simulink model "uz_3ph_ParameterID"  (R2022b)
settings: Solver=FixedStepDiscrete  StartTime=0.0  StopTime=160  FixedStep=0.000005  RelTol=1e-3  EnableMultiTasking=on
model workspace (MATLAB code in the model file):
  | cmdLim = Simulink.Parameter;
  | cmdLim.Value = 15;
  | cmdLim.Description = 'Limit for controlling the maximum surface command angle.';
  | cmdLim.Min = 0;
  | cmdLim.Max = 90;
  | cmdLim.DocUnits = 'deg';
  | 
  | dispGain = Simulink.Parameter;
  | dispGain.Value = 0.75;
  | dispGain.Description = 'Gain applied to the displacement error.';
  | dispGain.Min = 0;
  | dispGain.Max = [];
  | dispGain.DocUnits = 'deg/sec/deg';
  | 
  | dispLim = Simulink.Parameter;
  | dispLim.Value = 30;
  | dispLim.Description = 'Limit for controlling the maximum commanded angle.';
  | dispLim.Min = 0;
  | dispLim.Max = 180;
  | dispLim.DocUnits = 'deg';
  | 
  | intGain = Simulink.Parameter;
  | intGain.Value = 0.5;
  | intGain.Description = 'Gain applied to the integral error.';
  | intGain.Min = 0;
  | intGain.Max = [];
  | intGain.DocUnits = 'deg/sec/deg/sec';
  | 
  | intLim = Simulink.Parameter;
  | intLim.Value = 5;
  | intLim.Description = 'Limit for controlling the maximum commanded angle.';
  | intLim.Min = 0;
  | intLim.Max = 90;
  | intLim.DocUnits = 'deg';
  | 
  | rateGain = Simulink.Parameter;
  | rateGain.Value = 2;
  | rateGain.Description = 'Gain applied to the rate error.';
  | rateGain.Min = 0;
  | rateGain.Max = [];
  | rateGain.DocUnits = 'deg/deg/sec';
  | 
  | rateLim = Simulink.Parameter;
  | rateLim.Value = 6;
  | rateLim.Description = 'Limit for controlling the maximum commanded angle.';
  | rateLim.Min = 0;
  | rateLim.Max = 180;
  | rateLim.DocUnits = 'deg/sec';
  | 
  | hdgGain = Simulink.Parameter;
  | hdgGain.Value = 0.015;
values from neighbouring files (symbols this model uses):
  d_d_TMS = 0.005    [Parameter_Init_Buehler_201.m]
  d_f_hardware = 200000    [Parameter_Init_Buehler_201.m]
  d_f_states = 20000    [Parameter_Init_Buehler_201.m]
  d_i_max = 15    [Parameter_Init_Buehler_201.m]
  d_i_min = -d_i_max    (= -15)    [Parameter_Init_Buehler_201.m]
  d_I_n = 8    [Parameter_Init_Buehler_201.m]
  d_J_Coupling_M_E = 2e-6    (= 2e-06)    [Parameter_Init_Buehler_201.m]
  d_J_Coupling_M_Ms = 2e-20    [Parameter_Init_Buehler_201.m]
  d_J_Ms_L = d_J_Ms_M    (= 1.26363648e-05)    [Parameter_Init_Buehler_201.m]
  d_J_Ms_M = 0.5*0.5*((0.5*d_d_Ms)^4)*3.14*d_l_Ms*d_rho_Ms    (= 1.26363648e-05)    [Parameter_Init_Buehler_201.m]
  d_L_d = 0.00031    [Parameter_Init_Buehler_201.m]
  d_L_q = 0.00033    [Parameter_Init_Buehler_201.m]
  d_p = 4    [Parameter_Init_Buehler_201.m]
  d_psi_pm = 0.0075    [Parameter_Init_Buehler_201.m]
  d_R_ph = d_R_ph_ph/2    (= 0.089)    [Parameter_Init_Buehler_201.m]
  d_y_max = 10    [Parameter_Init_Buehler_201.m]
  d_y_min = -d_y_max    (= -10)    [Parameter_Init_Buehler_201.m]
undefined symbols (not defined in the file or in its folder): i_dq, i_dq_ref, n_ref, V_abc, v_dq
libraries: fl_lib x47, nesl_utility x30, ee_lib x18, simulink x8, spsabctodq0Lib x2, spsdq0toabcLib x1, spsTriangleGeneratorLib x1
(part 3 of 4)

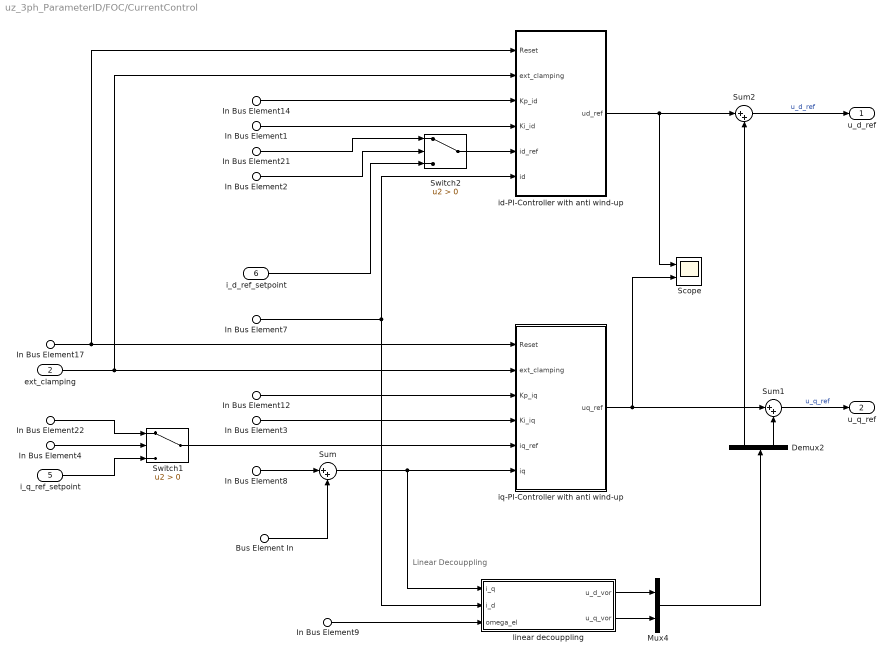
== system uz_3ph_ParameterID/FOC/CurrentControl ==
  note: Linear Decouppling
  Bus Element In : Inport  PortName=TwoMassID_output  Element=PRBS_out
  ext_clamping : Inport  Port=2
  In Bus Element1 : Inport  Port=3  PortName=FOC_State_outputs  Element=Ki_id_out
  In Bus Element14 : Inport  Port=3  PortName=FOC_State_outputs  Element=Kp_id_out
  In Bus Element2 : Inport  Port=3  PortName=FOC_State_outputs  Element=enableFOC_current
  In Bus Element4 : Inport  Port=3  PortName=FOC_State_outputs  Element=enableFOC_current
  In Bus Element21 : Inport  Port=3  PortName=FOC_State_outputs  Element=i_dq_ref.d
  In Bus Element22 : Inport  Port=3  PortName=FOC_State_outputs  Element=i_dq_ref.q
  In Bus Element17 : Inport  Port=3  PortName=FOC_State_outputs  Element=resetIntegrator
  In Bus Element12 : Inport  Port=3  PortName=FOC_State_outputs  Element=Kp_iq_out
  In Bus Element3 : Inport  Port=3  PortName=FOC_State_outputs  Element=Ki_iq_out
  In Bus Element9 : Inport  Port=4  PortName=ActualValues  Element=omega_el
  In Bus Element7 : Inport  Port=4  PortName=ActualValues  Element=i_dq.d
  In Bus Element8 : Inport  Port=4  PortName=ActualValues  Element=i_dq.q
  i_q_ref_setpoint : Inport  Port=5
  i_d_ref_setpoint : Inport  Port=6
  Demux2 : Demux  Outputs=2
  Mux4 : Mux  Inputs=2
  Scope : Scope  NumInputPorts=2
  Sum : Sum  Inputs=|++
  Sum1 : Sum  Inputs=|++
  Sum2 : Sum  Inputs=|++
  Switch1 : Switch  Criteria=u2 > Threshold  SaturateOnIntegerOverflow=off  InputSameDT=off
  Switch2 : Switch  Criteria=u2 > Threshold  SaturateOnIntegerOverflow=off  InputSameDT=off
  id-PI-Controller with anti wind-up : Subsystem
  iq-PI-Controller with anti wind-up : Subsystem
  linear decouppling : Subsystem
  u_d_ref : Outport  OutDataTypeStr=single
  u_q_ref : Outport  Port=2  OutDataTypeStr=single
  wires:
  In Bus Element7/1 -> id-PI-Controller with anti wind-up/6(id), linear decouppling/2(i_d)
  In Bus Element1/1 -> id-PI-Controller with anti wind-up/4(Ki_id)
  Sum/1 -> linear decouppling/1(i_q), iq-PI-Controller with anti wind-up/6(iq)
  In Bus Element3/1 -> iq-PI-Controller with anti wind-up/4(Ki_iq)
  In Bus Element14/1 -> id-PI-Controller with anti wind-up/3(Kp_id)
  In Bus Element12/1 -> iq-PI-Controller with anti wind-up/3(Kp_iq)
  In Bus Element17/1 -> iq-PI-Controller with anti wind-up/1(Reset), id-PI-Controller with anti wind-up/1(Reset)
  Switch1/1 -> iq-PI-Controller with anti wind-up/5(iq_ref)
  ext_clamping/1 -> iq-PI-Controller with anti wind-up/2(ext_clamping), id-PI-Controller with anti wind-up/2(ext_clamping)
  In Bus Element9/1 -> linear decouppling/3(omega_el)
  Mux4/1 -> Demux2/1
  linear decouppling/1(u_d_vor) -> Mux4/1
  linear decouppling/2(u_q_vor) -> Mux4/2
  Demux2/2 -> Sum1/2
  iq-PI-Controller with anti wind-up/1(uq_ref) -> Scope/2, Sum1/1
  id-PI-Controller with anti wind-up/1(ud_ref) -> Scope/1, Sum2/1
  Demux2/1 -> Sum2/2
  Sum1/1 -> u_q_ref/1  "u_q_ref"
  In Bus Element22/1 -> Switch1/1
  In Bus Element4/1 -> Switch1/2
  i_q_ref_setpoint/1 -> Switch1/3
  Sum2/1 -> u_d_ref/1  "u_d_ref"
  In Bus Element21/1 -> Switch2/1
  i_d_ref_setpoint/1 -> Switch2/3
  Switch2/1 -> id-PI-Controller with anti wind-up/5(id_ref)
  In Bus Element2/1 -> Switch2/2
  In Bus Element8/1 -> Sum/1
  Bus Element In/1 -> Sum/2

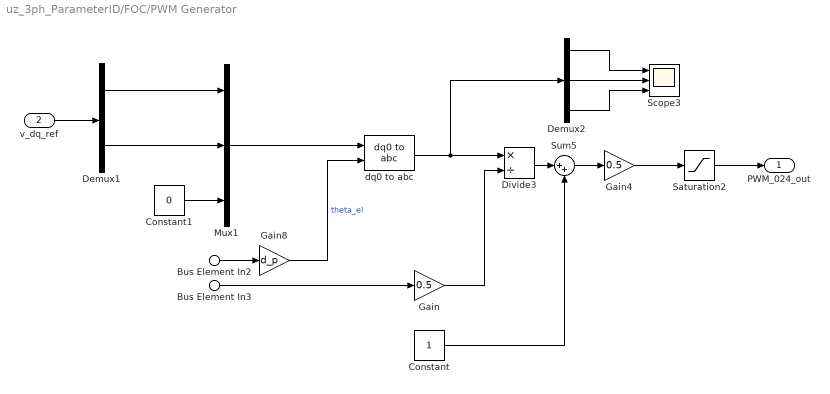
== system uz_3ph_ParameterID/FOC/PWM Generator ==
  Bus Element In2 : Inport  PortName=ActualValues  Element=theta_m
  Bus Element In3 : Inport  PortName=ActualValues  Element=V_DC
  v_dq_ref : Inport  Port=2
  Constant : Constant  OutDataTypeStr=single
  Constant1 : Constant  Value=0  OutDataTypeStr=single
  Demux1 : Demux  Outputs=2
  Demux2 : Demux  Outputs=3
  Divide3 : Product  Inputs=*/
  Gain : Gain  Gain=0.5
  Gain4 : Gain  Gain=0.5
  Gain8 : Gain  Gain=d_p  OutDataTypeStr=single
  Mux1 : Mux  Inputs=3
  Saturation2 : Saturate  UpperLimit=1  LowerLimit=0
  Scope3 : Scope  NumInputPorts=3
  Sum5 : Sum  Inputs=|++
  dq0 to abc : spsdq0toabcLib/dq0 to abc  Alignment=Aligned with phase A axis
  PWM_024_out : Outport  VectorParamsAs1DForOutWhenUnconnected=off
  wires:
  Constant/1 -> Sum5/2
  Demux2/2 -> Scope3/2
  Gain4/1 -> Saturation2/1
  Demux2/1 -> Scope3/1
  Demux2/3 -> Scope3/3
  Gain/1 -> Divide3/2
  Sum5/1 -> Gain4/1
  Mux1/1 -> dq0 to abc/1
  dq0 to abc/1 -> Demux2/1, Divide3/1
  Divide3/1 -> Sum5/1
  Bus Element In3/1 -> Gain/1
  Constant1/1 -> Mux1/3
  Demux1/2 -> Mux1/2
  Saturation2/1 -> PWM_024_out/1
  v_dq_ref/1 -> Demux1/1
  Demux1/1 -> Mux1/1
  Bus Element In2/1 -> Gain8/1
  Gain8/1 -> dq0 to abc/2  "theta_el"

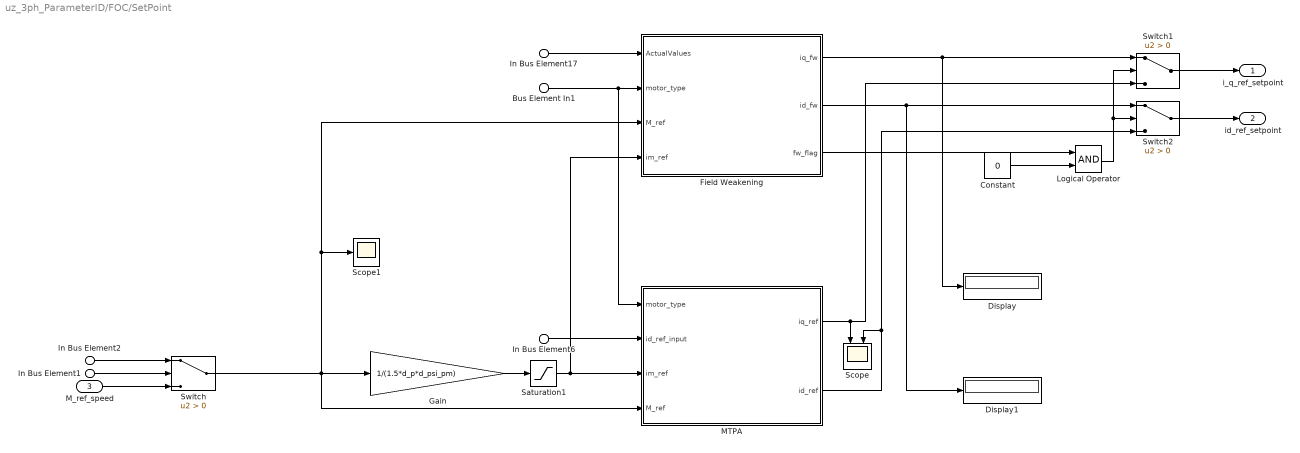
== system uz_3ph_ParameterID/FOC/SetPoint ==
  In Bus Element17 : Inport  PortName=ActualValues
  In Bus Element6 : Inport  Port=2  PortName=FOC_State_outputs  Element=i_dq_ref.d
  In Bus Element1 : Inport  Port=2  PortName=FOC_State_outputs  Element=enableFOC_torque
  In Bus Element2 : Inport  Port=2  PortName=FOC_State_outputs  Element=M_ref_FOC
  M_ref_speed : Inport  Port=3
  Bus Element In1 : Inport  Port=4  PortName=GlobalConfig  Element=motor_type
  Constant : Constant  Value=0
  Display : Display
  Display1 : Display
  Field Weakening : Subsystem
  Gain : Gain  Gain=1/(1.5*d_p*d_psi_pm)
  Logical Operator : Logic  AllPortsSameDT=off  OutDataTypeStr=boolean
  MTPA : Subsystem
  Saturation1 : Saturate  UpperLimit=d_i_max  LowerLimit=d_i_min
  Scope : Scope  NumInputPorts=2
  Scope1 : Scope
  Switch : Switch  Criteria=u2 > Threshold  SaturateOnIntegerOverflow=off  InputSameDT=off
  Switch1 : Switch  Criteria=u2 > Threshold  SaturateOnIntegerOverflow=off  InputSameDT=off
  Switch2 : Switch  Criteria=u2 > Threshold  SaturateOnIntegerOverflow=off  InputSameDT=off
  i_q_ref_setpoint : Outport  OutDataTypeStr=single
  id_ref_setpoint : Outport  Port=2  OutDataTypeStr=single
  wires:
  In Bus Element17/1 -> Field Weakening/1(ActualValues)
  Bus Element In1/1 -> MTPA/1(motor_type), Field Weakening/2(motor_type)
  In Bus Element6/1 -> MTPA/2(id_ref_input)
  MTPA/1(iq_ref) -> Switch1/3, Scope/1
  MTPA/2(id_ref) -> Switch2/3, Scope/2
  Switch2/1 -> id_ref_setpoint/1
  Field Weakening/2(id_fw) -> Display1/1, Switch2/1
  Saturation1/1 -> Field Weakening/4(im_ref), MTPA/3(im_ref)
  Field Weakening/1(iq_fw) -> Switch1/1, Display/1
  Logical Operator/1 -> Switch1/2, Switch2/2
  Gain/1 -> Saturation1/1
  Switch/1 -> Scope1/1, Field Weakening/3(M_ref), MTPA/4(M_ref), Gain/1
  Switch1/1 -> i_q_ref_setpoint/1
  Field Weakening/3(fw_flag) -> Logical Operator/1
  Constant/1 -> Logical Operator/2
  M_ref_speed/1 -> Switch/3
  In Bus Element1/1 -> Switch/2
  In Bus Element2/1 -> Switch/1

== system uz_3ph_ParameterID/FOC/SpeedControl ==
  ext_clamping : Inport
  In Bus Element7 : Inport  Port=2  PortName=FOC_State_outputs  Element=n_ref_FOC
  In Bus Element10 : Inport  Port=2  PortName=FOC_State_outputs  Element=resetIntegrator
  In Bus Element17 : Inport  Port=3  PortName=ActualValues  Element=omega_el
  Bus Element In1 : Inport  Port=4  PortName=GlobalConfig  Element=Ki_n
  Bus Element In : Inport  Port=4  PortName=GlobalConfig  Element=Kp_n
  Constant : Constant
  Constant1 : Constant  Value=-1
  Gain : Gain  Gain=1/d_p
  omega-PI-Controller with anti wind-up : Subsystem
  M_ref : Outport  OutDataTypeStr=single
  wires:
  In Bus Element10/1 -> omega-PI-Controller with anti wind-up/1(Reset)
  In Bus Element7/1 -> omega-PI-Controller with anti wind-up/5(n_ref_rpm)
  Bus Element In1/1 -> omega-PI-Controller with anti wind-up/4(Ki_n)
  Bus Element In/1 -> omega-PI-Controller with anti wind-up/3(Kp_n)
  ext_clamping/1 -> omega-PI-Controller with anti wind-up/2(ext_clamping)
  In Bus Element17/1 -> Gain/1
  omega-PI-Controller with anti wind-up/1(M_ref) -> M_ref/1
  Constant/1 -> omega-PI-Controller with anti wind-up/7(upper_limit)
  Constant1/1 -> omega-PI-Controller with anti wind-up/8(lower_limit)
  Gain/1 -> omega-PI-Controller with anti wind-up/6(omega)

== system uz_3ph_ParameterID/Hardware/Coupling Encoder ==
  note: 1) Add Subsystem or Model blocks as valid variant choices.
      | 2) You cannot connect blocks at this level. At simulation, connectivity is automatically
      | determined, based on the active variant and port name matching.
  Inertia : Subsystem  VariantControl=(default)
  Spring Damper System : Subsystem  VariantControl=TMS1
  Input : PMIOPort  Side=Left
  output : PMIOPort  Port=2  Side=Right

== system uz_3ph_ParameterID/Hardware/Measurement Shaft ==
  note: 1) Add Subsystem or Model blocks as valid variant choices.
      | 2) You cannot connect blocks at this level. At simulation, connectivity is automatically
      | determined, based on the active variant and port name matching.
  Spring Damper System : Subsystem  VariantControl=TMS1
  default : Subsystem  VariantControl=(default)
  Input : PMIOPort  Side=Left
  output : PMIOPort  Port=2  Side=Right

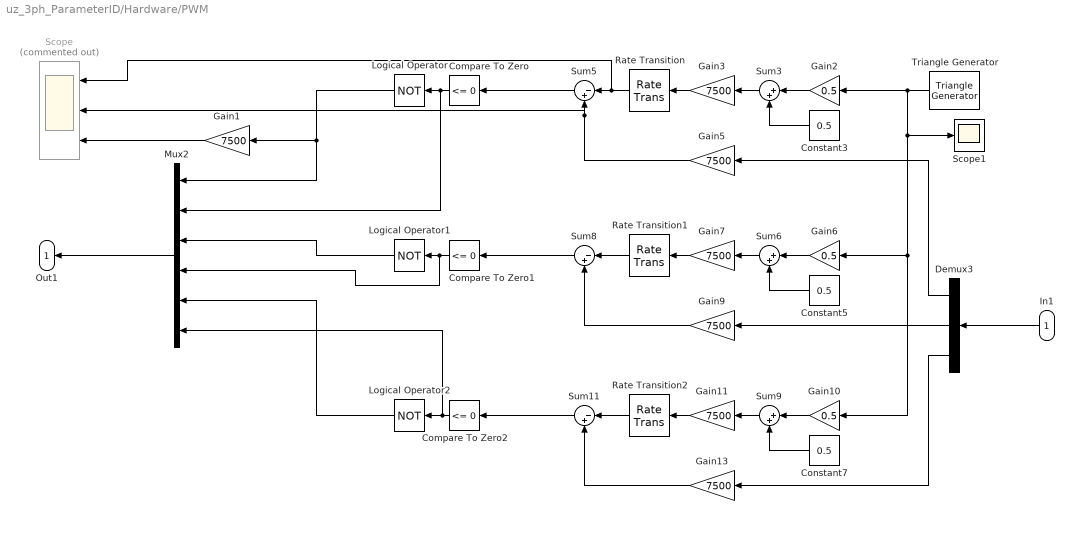
== system uz_3ph_ParameterID/Hardware/PWM ==
  In1 : Inport
  Compare To Zero : simulink/Logic and Bit Operations/Compare To Zero  relop=<=  OutDataTypeStr=boolean
  Compare To Zero1 : simulink/Logic and Bit Operations/Compare To Zero  relop=<=  OutDataTypeStr=boolean
  Compare To Zero2 : simulink/Logic and Bit Operations/Compare To Zero  relop=<=  OutDataTypeStr=boolean
  Constant3 : Constant  Value=0.5
  Constant5 : Constant  Value=0.5
  Constant7 : Constant  Value=0.5
  Demux3 : Demux  Outputs=3
  Gain{1,3,5,7,9,11,13} (7 alike) : Gain  Gain=7500  ParamDataTypeStr=single
  Gain10 : Gain  Gain=0.5
  Gain2 : Gain  Gain=0.5
  Gain6 : Gain  Gain=0.5
  Logical Operator : Logic  Operator=NOT  AllPortsSameDT=off  OutDataTypeStr=boolean
  Logical Operator1 : Logic  Operator=NOT  AllPortsSameDT=off  OutDataTypeStr=boolean
  Logical Operator2 : Logic  Operator=NOT  AllPortsSameDT=off  OutDataTypeStr=boolean
  Mux2 : Mux  Inputs=6
  Rate Transition : RateTransition  OutPortSampleTime=1/d_f_hardware
  Rate Transition1 : RateTransition  OutPortSampleTime=1/d_f_hardware
  Rate Transition2 : RateTransition  OutPortSampleTime=1/d_f_hardware
  Scope : Scope  Commented=on  NumInputPorts=3
  Scope1 : Scope
  Sum11 : Sum  Inputs=|-+
  Sum3 : Sum  Inputs=|++
  Sum5 : Sum  Inputs=|-+
  Sum6 : Sum  Inputs=|++
  Sum8 : Sum  Inputs=|-+
  Sum9 : Sum  Inputs=|++
  Triangle Generator : spsTriangleGeneratorLib/Triangle Generator  Freq=10000  Phase=0  Ts=1/d_f_hardware
  Out1 : Outport  VectorParamsAs1DForOutWhenUnconnected=off
  wires:
  Demux3/3 -> Gain13/1
  Logical Operator2/1 -> Mux2/5
  Logical Operator1/1 -> Mux2/3
  Mux2/1 -> Out1/1
  Compare To Zero2/1 -> Mux2/6, Logical Operator2/1
  Gain10/1 -> Sum9/1
  Sum8/1 -> Compare To Zero1/1
  Gain6/1 -> Sum6/1
  Sum9/1 -> Gain11/1
  Triangle Generator/1 -> Scope1/1, Gain10/1, Gain6/1, Gain2/1
  Sum6/1 -> Gain7/1
  Demux3/2 -> Gain9/1
  Compare To Zero1/1 -> Mux2/4, Logical Operator1/1
  Constant5/1 -> Sum6/2
  Constant7/1 -> Sum9/2
  Sum11/1 -> Compare To Zero2/1
  Sum3/1 -> Gain3/1
  Constant3/1 -> Sum3/2
  Demux3/1 -> Gain5/1
  Sum5/1 -> Compare To Zero/1
  Gain2/1 -> Sum3/1
  In1/1 -> Demux3/1
  Gain3/1 -> Rate Transition/1
  Gain7/1 -> Rate Transition1/1
  Gain11/1 -> Rate Transition2/1
  Gain5/1 -> Scope/2, Sum5/2
  Gain9/1 -> Sum8/2
  Gain13/1 -> Sum11/2
  Rate Transition/1 -> Scope/1, Sum5/1
  Rate Transition1/1 -> Sum8/1
  Rate Transition2/1 -> Sum11/1
  Logical Operator/1 -> Gain1/1, Mux2/1
  Compare To Zero/1 -> Mux2/2, Logical Operator/1
  Gain1/1 -> Scope/3

== system uz_3ph_ParameterID/Hardware/Switch f. TMS ==
  note: 1) Add Subsystem or Model blocks as valid variant choices.
      | 2) You cannot connect blocks at this level. At simulation, connectivity is automatically
      | determined, based on the active variant and port name matching.
  closed : Subsystem  VariantControl=d_KupplZus==1
  open : Subsystem  VariantControl=d_KupplZus==0
  Input : PMIOPort  Side=Left
  output : PMIOPort  Port=2  Side=Right

== system uz_3ph_ParameterID/Hardware/coupling m. shaft ==
  note: 1) Add Subsystem or Model blocks as valid variant choices.
      | 2) You cannot connect blocks at this level. At simulation, connectivity is automatically
      | determined, based on the active variant and port name matching.
  Inertia : Subsystem  VariantControl=(default)
  Spring Damper System : Subsystem  VariantControl=TMS1
  Input : PMIOPort  Side=Left
  output : PMIOPort  Port=2  Side=Right

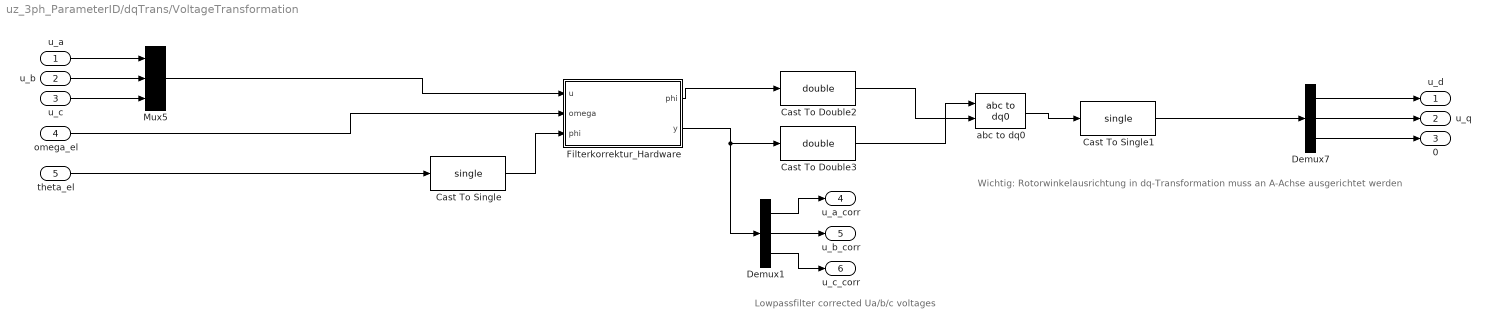
== system uz_3ph_ParameterID/dqTrans/VoltageTransformation ==
  note: Lowpassfilter corrected Ua/b/c voltages
  note: Wichtig: Rotorwinkelausrichtung in dq-Transformation
      | muss an A-Achse ausgerichtet werden
  u_a : Inport
  u_b : Inport  Port=2
  u_c : Inport  Port=3
  omega_el : Inport  Port=4
  theta_el : Inport  Port=5
  Cast To Double2 : DataTypeConversion  OutDataTypeStr=double  SaturateOnIntegerOverflow=off  RndMeth=Floor
  Cast To Double3 : DataTypeConversion  OutDataTypeStr=double  SaturateOnIntegerOverflow=off  RndMeth=Floor
  Cast To Single : DataTypeConversion  OutDataTypeStr=single  SaturateOnIntegerOverflow=off  RndMeth=Floor
  Cast To Single1 : DataTypeConversion  OutDataTypeStr=single  SaturateOnIntegerOverflow=off  RndMeth=Floor
  Demux1 : Demux  Outputs=3
  Demux7 : Demux  Outputs=3
  Filterkorrektur_Hardware : MATLAB Function  TreatAsAtomicUnit=on
  Mux5 : Mux  Inputs=3
  abc to dq0 : spsabctodq0Lib/abc to dq0  Alignment=Aligned with phase A axis
  u_d : Outport  VectorParamsAs1DForOutWhenUnconnected=off
  u_q : Outport  Port=2  VectorParamsAs1DForOutWhenUnconnected=off
  0 : Outport  Port=3  VectorParamsAs1DForOutWhenUnconnected=off
  u_a_corr : Outport  Port=4  VectorParamsAs1DForOutWhenUnconnected=off
  u_b_corr : Outport  Port=5  VectorParamsAs1DForOutWhenUnconnected=off
  u_c_corr : Outport  Port=6  VectorParamsAs1DForOutWhenUnconnected=off
  wires:
  abc to dq0/1 -> Cast To Single1/1
  Cast To Single1/1 -> Demux7/1
  Cast To Double3/1 -> abc to dq0/1
  Filterkorrektur_Hardware/2(y) -> Demux1/1, Cast To Double3/1
  Cast To Double2/1 -> abc to dq0/2
  Filterkorrektur_Hardware/1(phi) -> Cast To Double2/1
  Demux7/2 -> u_q/1
  Demux7/3 -> 0/1
  u_b/1 -> Mux5/2
  u_c/1 -> Mux5/3
  u_a/1 -> Mux5/1
  omega_el/1 -> Filterkorrektur_Hardware/2(omega)
  Mux5/1 -> Filterkorrektur_Hardware/1(u)
  theta_el/1 -> Cast To Single/1
  Cast To Single/1 -> Filterkorrektur_Hardware/3("phi ")
  Demux7/1 -> u_d/1
  Demux1/1 -> u_a_corr/1
  Demux1/2 -> u_b_corr/1
  Demux1/3 -> u_c_corr/1

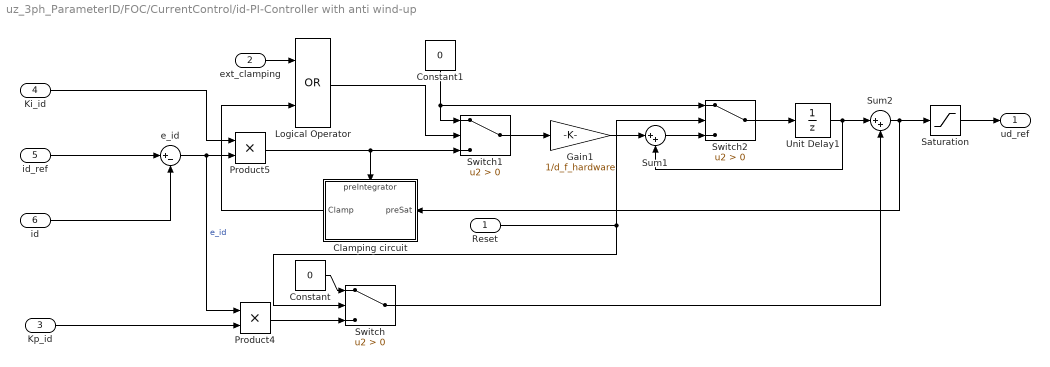
== system uz_3ph_ParameterID/FOC/CurrentControl/id-PI-Controller with anti wind-up ==
  Reset : Inport
  ext_clamping : Inport  Port=2
  Kp_id : Inport  Port=3
  Ki_id : Inport  Port=4
  id_ref : Inport  Port=5
  id : Inport  Port=6
  Clamping circuit : Subsystem
      settings: PortSchema="{\"entries\":[{\"content\":{\"sides\":[{\"content\":{\"connectorIds\":[\"In1\"]},\"type\":\"ConnectorPlacement.EquallySpacedRectSide\",\"uuid\":\"9b5eb3d3-336d-4b55-a615-0420b1cf4a48\"},{\"content\":{\"connectorIds\":[\"Out1\"],\"side\":\"RIGHT\"},\"type\":\"ConnectorPlacement.EquallySpacedRectSide\",\"uuid\":\"a73559ab-79dd-4c84-b45a-6a43ba4812e9\"},{\"content\":{\"connectorIds\":[\"In2\"],\"side\":\"TOP\"},\"type\":\"ConnectorPlacement.EquallySpacedRectSide\",\"uuid\":\"82c30f31-c271-4a2b-89be-8686aa9e20f3\"}]},\"type\":\"ConnectorPlacement.EquallySpacedConnector\",\"uuid\":\"376d2fe4-39b3-495b-8d80-8756076e2730\"}],\"packageUris\":[\"http://schema.mathworks.com/mf0/Connector/R2020b\"],\"version\":\"1.0\"}"
  Constant : Constant  Value=0  SampleTime=1/d_f_hardware
  Constant1 : Constant  Value=0  SampleTime=1/d_f_hardware
  Gain1 : Gain  Gain=1/d_f_hardware
  Logical Operator : Logic  Operator=OR  AllPortsSameDT=off  OutDataTypeStr=boolean
  Product4 : Product
  Product5 : Product
  Saturation : Saturate  UpperLimit=d_y_max  LowerLimit=d_y_min
  Sum1 : Sum  Inputs=|++  OutDataTypeStr=single
  Sum2 : Sum  Inputs=|++  OutDataTypeStr=single
  Switch : Switch  Criteria=u2 > Threshold  SaturateOnIntegerOverflow=off  InputSameDT=off
  Switch1 : Switch  Criteria=u2 > Threshold  SaturateOnIntegerOverflow=off  InputSameDT=off
  Switch2 : Switch  Criteria=u2 > Threshold  SaturateOnIntegerOverflow=off  InputSameDT=off
  Unit Delay1 : UnitDelay  SampleTime=-1  HasFrameUpgradeWarning=on
  e_id : Sum  Inputs=|+-
  ud_ref : Outport
  wires:
  Unit Delay1/1 -> Sum2/1, Sum1/2
  Kp_id/1 -> Product4/2
  id_ref/1 -> e_id/1
  Ki_id/1 -> Product5/1
  id/1 -> e_id/2
  e_id/1 -> Product5/2, Product4/1  "e_id"
  Switch/1 -> Sum2/2
  Logical Operator/1 -> Switch1/2
  ext_clamping/1 -> Logical Operator/1
  Sum2/1 -> Saturation/1, Clamping circuit/1(preSat)
  Clamping circuit/1(Clamp) -> Logical Operator/2
  Product5/1 -> Switch1/3, Clamping circuit/2(preIntegrator)
  Saturation/1 -> ud_ref/1
  Constant/1 -> Switch/1
  Product4/1 -> Switch/3
  Gain1/1 -> Sum1/1
  Constant1/1 -> Switch2/1, Switch1/1
  Reset/1 -> Switch/2, Switch2/2
  Sum1/1 -> Switch2/3
  Switch2/1 -> Unit Delay1/1
  Switch1/1 -> Gain1/1

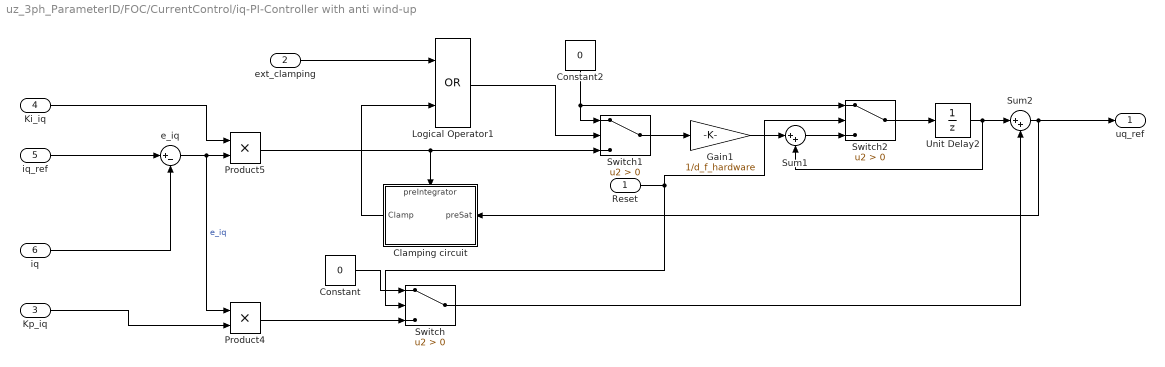
== system uz_3ph_ParameterID/FOC/CurrentControl/iq-PI-Controller with anti wind-up ==
  Reset : Inport
  ext_clamping : Inport  Port=2
  Kp_iq : Inport  Port=3
  Ki_iq : Inport  Port=4
  iq_ref : Inport  Port=5
  iq : Inport  Port=6
  Clamping circuit : Subsystem
      settings: PortSchema="{\"entries\":[{\"content\":{\"sides\":[{\"content\":{\"connectorIds\":[\"In1\"]},\"type\":\"ConnectorPlacement.EquallySpacedRectSide\",\"uuid\":\"9b5eb3d3-336d-4b55-a615-0420b1cf4a48\"},{\"content\":{\"connectorIds\":[\"Out1\"],\"side\":\"RIGHT\"},\"type\":\"ConnectorPlacement.EquallySpacedRectSide\",\"uuid\":\"a73559ab-79dd-4c84-b45a-6a43ba4812e9\"},{\"content\":{\"connectorIds\":[\"In2\"],\"side\":\"TOP\"},\"type\":\"ConnectorPlacement.EquallySpacedRectSide\",\"uuid\":\"82c30f31-c271-4a2b-89be-8686aa9e20f3\"}]},\"type\":\"ConnectorPlacement.EquallySpacedConnector\",\"uuid\":\"376d2fe4-39b3-495b-8d80-8756076e2730\"}],\"packageUris\":[\"http://schema.mathworks.com/mf0/Connector/R2020b\"],\"version\":\"1.0\"}"
  Constant : Constant  Value=0  SampleTime=1/d_f_hardware
  Constant2 : Constant  Value=0  SampleTime=1/d_f_hardware
  Gain1 : Gain  Gain=1/d_f_hardware
  Logical Operator1 : Logic  Operator=OR  AllPortsSameDT=off  OutDataTypeStr=boolean
  Product4 : Product
  Product5 : Product
  Sum1 : Sum  Inputs=|++  OutDataTypeStr=single
  Sum2 : Sum  Inputs=|++  OutDataTypeStr=single
  Switch : Switch  Criteria=u2 > Threshold  SaturateOnIntegerOverflow=off  InputSameDT=off
  Switch1 : Switch  Criteria=u2 > Threshold  SaturateOnIntegerOverflow=off  InputSameDT=off
  Switch2 : Switch  Criteria=u2 > Threshold  SaturateOnIntegerOverflow=off  InputSameDT=off
  Unit Delay2 : UnitDelay  SampleTime=-1  HasFrameUpgradeWarning=on
  e_iq : Sum  Inputs=|+-
  uq_ref : Outport
  wires:
  ext_clamping/1 -> Logical Operator1/1
  Kp_iq/1 -> Product4/2
  Ki_iq/1 -> Product5/1
  iq_ref/1 -> e_iq/1
  iq/1 -> e_iq/2
  e_iq/1 -> Product5/2, Product4/1  "e_iq"
  Unit Delay2/1 -> Sum2/1, Sum1/2
  Clamping circuit/1(Clamp) -> Logical Operator1/2
  Sum2/1 -> uq_ref/1, Clamping circuit/1(preSat)
  Switch/1 -> Sum2/2
  Constant/1 -> Switch/1
  Product4/1 -> Switch/3
  Switch2/1 -> Unit Delay2/1
  Gain1/1 -> Sum1/1
  Constant2/1 -> Switch2/1, Switch1/1
  Sum1/1 -> Switch2/3
  Product5/1 -> Switch1/3, Clamping circuit/2(preIntegrator)
  Switch1/1 -> Gain1/1
  Reset/1 -> Switch2/2, Switch/2
  Logical Operator1/1 -> Switch1/2

== system uz_3ph_ParameterID/FOC/CurrentControl/linear decouppling ==
  i_q : Inport
  i_d : Inport  Port=2
  omega_el : Inport  Port=3
  Gain : Gain  Gain=-d_L_q
  Gain4 : Gain  Gain=d_L_d
  Product : Product  SaturateOnIntegerOverflow=on
  Product1 : Product  SaturateOnIntegerOverflow=on
  Sum : Sum  Inputs=|++
  d_psi_pm : Constant  Value=d_psi_pm  OutDataTypeStr=Inherit: Inherit via back propagation  SampleTime=1/d_f_hardware
  u_d_vor : Outport  VectorParamsAs1DForOutWhenUnconnected=off
  u_q_vor : Outport  Port=2  VectorParamsAs1DForOutWhenUnconnected=off
  wires:
  i_q/1 -> Product/1
  Product1/1 -> u_q_vor/1
  Gain/1 -> Product/2
  Sum/1 -> Product1/1
  Product/1 -> u_d_vor/1
  omega_el/1 -> Gain/1, Product1/2
  Gain4/1 -> Sum/1
  d_psi_pm/1 -> Sum/2
  i_d/1 -> Gain4/1

== system uz_3ph_ParameterID/FOC/SetPoint/Field Weakening ==
  ActualValues : Inport  OutDataTypeStr=Bus: uz_ParaID_ActualValues_t
  motor_type : Inport  Port=2  OutDataTypeStr=uint16
  M_ref : Inport  Port=3  OutDataTypeStr=single
  im_ref : Inport  Port=4  OutDataTypeStr=single
  Constant : Constant  Value=d_R_ph  OutDataTypeStr=single
  Constant1 : Constant  Value=d_L_q  OutDataTypeStr=single
  Constant2 : Constant  Value=d_L_d  OutDataTypeStr=single
  Constant3 : Constant  Value=d_psi_pm  OutDataTypeStr=single
  Constant4 : Constant  Value=d_i_max  OutDataTypeStr=single
  Constant5 : Constant  Value=d_p  OutDataTypeStr=single
  Gain : Gain  Gain=60/(2*d_p*pi)
  MATLAB Function : MATLAB Function  TreatAsAtomicUnit=on
  n_cut in rpm : Display
  iq_fw : Outport  OutDataTypeStr=single
  id_fw : Outport  Port=2  OutDataTypeStr=single
  fw_flag : Outport  Port=3  OutDataTypeStr=boolean
  wires:
  Constant4/1 -> MATLAB Function/1(I_max)
  ActualValues/1 -> MATLAB Function/2(ActualValues)
  Constant/1 -> MATLAB Function/3(R)
  Constant1/1 -> MATLAB Function/4(Lq)
  Constant2/1 -> MATLAB Function/5(Ld)
  Constant3/1 -> MATLAB Function/6(psi_pm)
  MATLAB Function/2(iq_fw) -> iq_fw/1
  MATLAB Function/1(id_fw) -> id_fw/1
  motor_type/1 -> MATLAB Function/7(motor_type)
  MATLAB Function/3(fw_flag) -> fw_flag/1
  M_ref/1 -> MATLAB Function/9(M_ref)
  im_ref/1 -> MATLAB Function/10(im_ref)
  Constant5/1 -> MATLAB Function/8(polepairs)
  MATLAB Function/4(omega_cut) -> Gain/1
  Gain/1 -> n_cut in rpm/1

== system uz_3ph_ParameterID/FOC/SetPoint/MTPA ==
  motor_type : Inport  OutDataTypeStr=uint16
  id_ref_input : Inport  Port=2  OutDataTypeStr=single
  im_ref : Inport  Port=3  OutDataTypeStr=single
  M_ref : Inport  Port=4  OutDataTypeStr=single
  Constant1 : Constant  Value=d_L_q  OutDataTypeStr=single
  Constant2 : Constant  Value=d_L_d  OutDataTypeStr=single
  Constant3 : Constant  Value=d_psi_pm  OutDataTypeStr=single
  Constant4 : Constant  Value=d_i_max  OutDataTypeStr=single
  Constant5 : Constant  Value=d_p  OutDataTypeStr=single
  MATLAB Function : MATLAB Function  TreatAsAtomicUnit=on
  Saturation : Saturate  UpperLimit=d_i_max  LowerLimit=d_i_min
  iq_ref : Outport  OutDataTypeStr=single
  id_ref : Outport  Port=2  OutDataTypeStr=single
  wires:
  Constant4/1 -> MATLAB Function/1(I_max)
  Constant1/1 -> MATLAB Function/4(Lq)
  Constant2/1 -> MATLAB Function/5(Ld)
  Constant3/1 -> MATLAB Function/6(psi_pm)
  MATLAB Function/2(id_ref) -> id_ref/1
  MATLAB Function/1(iq_ref) -> iq_ref/1
  id_ref_input/1 -> Saturation/1
  Saturation/1 -> MATLAB Function/8(id_ref_input)
  im_ref/1 -> MATLAB Function/2(im_ref)
  motor_type/1 -> MATLAB Function/9(motor_type)
  Constant5/1 -> MATLAB Function/7(polepairs)
  M_ref/1 -> MATLAB Function/3(M_ref)

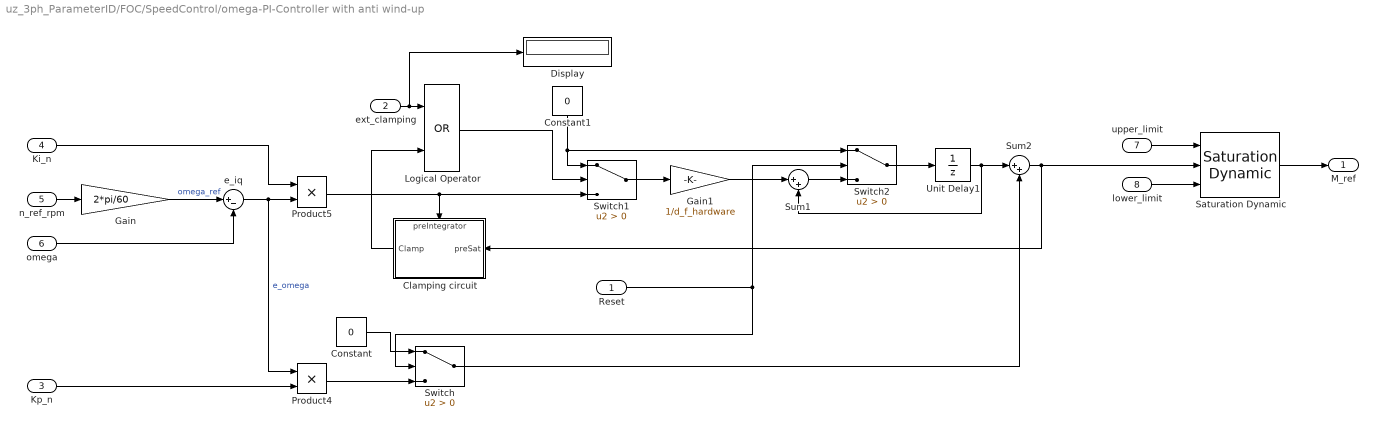
== system uz_3ph_ParameterID/FOC/SpeedControl/omega-PI-Controller with anti wind-up ==
  Reset : Inport
  ext_clamping : Inport  Port=2
  Kp_n : Inport  Port=3
  Ki_n : Inport  Port=4
  n_ref_rpm : Inport  Port=5
  omega : Inport  Port=6
  upper_limit : Inport  Port=7
  lower_limit : Inport  Port=8
  Clamping circuit : Subsystem
      settings: PortSchema="{\"entries\":[{\"content\":{\"sides\":[{\"content\":{\"connectorIds\":[\"In1\"]},\"type\":\"ConnectorPlacement.EquallySpacedRectSide\",\"uuid\":\"9b5eb3d3-336d-4b55-a615-0420b1cf4a48\"},{\"content\":{\"connectorIds\":[\"Out1\"],\"side\":\"RIGHT\"},\"type\":\"ConnectorPlacement.EquallySpacedRectSide\",\"uuid\":\"a73559ab-79dd-4c84-b45a-6a43ba4812e9\"},{\"content\":{\"connectorIds\":[\"In2\"],\"side\":\"TOP\"},\"type\":\"ConnectorPlacement.EquallySpacedRectSide\",\"uuid\":\"82c30f31-c271-4a2b-89be-8686aa9e20f3\"}]},\"type\":\"ConnectorPlacement.EquallySpacedConnector\",\"uuid\":\"376d2fe4-39b3-495b-8d80-8756076e2730\"}],\"packageUris\":[\"http://schema.mathworks.com/mf0/Connector/R2020b\"],\"version\":\"1.0\"}"
  Constant : Constant  Value=0  SampleTime=1/d_f_hardware
  Constant1 : Constant  Value=0  SampleTime=1/d_f_hardware
  Display : Display
  Gain : Gain  Gain=2*pi/60
  Gain1 : Gain  Gain=1/d_f_hardware
  Logical Operator : Logic  Operator=OR  AllPortsSameDT=off  OutDataTypeStr=boolean
  Product4 : Product
  Product5 : Product
  Saturation Dynamic : simulink/Discontinuities/Saturation Dynamic  OutMin=[]  OutMax=[]  OutDataTypeStr=Inherit: Same as second input  OutDataType=fixdt(1, 16)  OutScaling=2^-10  DoSatur=off
  Sum1 : Sum  Inputs=|++  OutDataTypeStr=single
  Sum2 : Sum  Inputs=|++  OutDataTypeStr=single
  Switch : Switch  Criteria=u2 > Threshold  SaturateOnIntegerOverflow=off  InputSameDT=off
  Switch1 : Switch  Criteria=u2 > Threshold  SaturateOnIntegerOverflow=off  InputSameDT=off
  Switch2 : Switch  Criteria=u2 > Threshold  OutDataTypeStr=single  SaturateOnIntegerOverflow=off  InputSameDT=off
  Unit Delay1 : UnitDelay  SampleTime=-1  HasFrameUpgradeWarning=on
  e_iq : Sum  Inputs=|+-  OutDataTypeStr=single
  M_ref : Outport
  wires:
  Kp_n/1 -> Product4/2
  Ki_n/1 -> Product5/1
  Gain/1 -> e_iq/1  "omega_ref"
  omega/1 -> e_iq/2
  e_iq/1 -> Product5/2, Product4/1  "e_omega"
  Switch/1 -> Sum2/2
  Unit Delay1/1 -> Sum2/1, Sum1/2
  Sum2/1 -> Clamping circuit/1(preSat), Saturation Dynamic/2
  ext_clamping/1 -> Display/1, Logical Operator/1
  Product5/1 -> Switch1/3, Clamping circuit/2(preIntegrator)
  Clamping circuit/1(Clamp) -> Logical Operator/2
  Constant/1 -> Switch/1
  Reset/1 -> Switch/2, Switch2/2
  Product4/1 -> Switch/3
  Constant1/1 -> Switch2/1, Switch1/1
  Logical Operator/1 -> Switch1/2
  n_ref_rpm/1 -> Gain/1
  Switch1/1 -> Gain1/1
  Gain1/1 -> Sum1/1
  Switch2/1 -> Unit Delay1/1
  Sum1/1 -> Switch2/3
  Saturation Dynamic/1 -> M_ref/1
  upper_limit/1 -> Saturation Dynamic/1
  lower_limit/1 -> Saturation Dynamic/3

== system uz_3ph_ParameterID/Hardware/Coupling Encoder/Inertia ==
  Trägheitsmoment3 : fl_lib/Mechanical/Rotational Elements/Inertia  Commented=on  inertia=d_J_Coupling_M_E kg*m^2  num_ports=foundation.enum.numPorts2.one  w_specify=off  w_priority=High  w=0 rad/s  w_nominal_specify=off  w_nominal_unit=rad/s  w_nominal_value=1  t_specify=off  t_priority=None  t=0 N*m  t_nominal_specify=off  t_nominal_unit=N*m  t_nominal_value=1
      settings: AttributesFormatString=J in [%<inertia_unit>]
  Input : PMIOPort  Side=Left
  output : PMIOPort  Port=2  Side=Right
  connections:
  Input/RConn1 -- Trägheitsmoment3/LConn1 -- output/RConn1

== system uz_3ph_ParameterID/Hardware/Coupling Encoder/Spring Damper System ==
  Rotational Spring : fl_lib/Mechanical/Rotational Elements/Rotational Spring  spr_rate=d_c_Coupling_M_E N*m/rad  w_specify=off  w_priority=None  w=0 rad/s  w_nominal_specify=off  w_nominal_unit=rad/s  w_nominal_value=1  t_specify=off  t_priority=None  t=0 N*m  t_nominal_specify=off  t_nominal_unit=N*m  t_nominal_value=1  phi_specify=off  phi_priority=High  phi=0 rad  phi_nominal_specify=off  phi_nominal_unit=rad  phi_nominal_value=1
  Trägheitsmoment1 : fl_lib/Mechanical/Rotational Elements/Inertia  inertia=d_J_Coupling_M_E/2 kg*m^2  num_ports=foundation.enum.numPorts2.one  w_specify=off  w_priority=High  w=0 rad/s  w_nominal_specify=off  w_nominal_unit=rad/s  w_nominal_value=1  t_specify=off  t_priority=None  t=0 N*m  t_nominal_specify=off  t_nominal_unit=N*m  t_nominal_value=1
      settings: AttributesFormatString=J in [%<inertia_unit>]
  Trägheitsmoment3 : fl_lib/Mechanical/Rotational Elements/Inertia  inertia=d_J_Coupling_M_E/2 kg*m^2  num_ports=foundation.enum.numPorts2.one  w_specify=off  w_priority=High  w=0 rad/s  w_nominal_specify=off  w_nominal_unit=rad/s  w_nominal_value=1  t_specify=off  t_priority=None  t=0 N*m  t_nominal_specify=off  t_nominal_unit=N*m  t_nominal_value=1
      settings: AttributesFormatString=J in [%<inertia_unit>]
  dm : fl_lib/Mechanical/Rotational Elements/Rotational Damper  Commented=on  D=0 N*m/(rad/s)  w_specify=off  w_priority=None  w=0 rad/s  w_nominal_specify=off  w_nominal_unit=rad/s  w_nominal_value=1  t_specify=off  t_priority=None  t=0 N*m  t_nominal_specify=off  t_nominal_unit=N*m  t_nominal_value=1
  Input : PMIOPort  Side=Left
  output : PMIOPort  Port=2  Side=Right
  connections:
  Rotational Spring/LConn1 -- dm/LConn1 -- Input/RConn1 -- Trägheitsmoment3/LConn1
  Trägheitsmoment1/LConn1 -- Rotational Spring/RConn1 -- dm/RConn1 -- output/RConn1

== system uz_3ph_ParameterID/Hardware/Measurement Shaft/Spring Damper System ==
  Rotational Spring : fl_lib/Mechanical/Rotational Elements/Rotational Spring  spr_rate=d_c_Ms N*m/rad  w_specify=off  w_priority=None  w=0 rad/s  w_nominal_specify=off  w_nominal_unit=rad/s  w_nominal_value=1  t_specify=off  t_priority=None  t=0 N*m  t_nominal_specify=off  t_nominal_unit=N*m  t_nominal_value=1  phi_specify=off  phi_priority=High  phi=0 rad  phi_nominal_specify=off  phi_nominal_unit=rad  phi_nominal_value=1
  Trägheitsmoment1 : fl_lib/Mechanical/Rotational Elements/Inertia  inertia=d_J_Ms_L kg*m^2  num_ports=foundation.enum.numPorts2.one  w_specify=off  w_priority=High  w=0 rad/s  w_nominal_specify=off  w_nominal_unit=rad/s  w_nominal_value=1  t_specify=off  t_priority=None  t=0 N*m  t_nominal_specify=off  t_nominal_unit=N*m  t_nominal_value=1
      settings: AttributesFormatString=J in [%<inertia_unit>]
  Trägheitsmoment3 : fl_lib/Mechanical/Rotational Elements/Inertia  inertia=d_J_Ms_M kg*m^2  num_ports=foundation.enum.numPorts2.one  w_specify=off  w_priority=High  w=0 rad/s  w_nominal_specify=off  w_nominal_unit=rad/s  w_nominal_value=1  t_specify=off  t_priority=None  t=0 N*m  t_nominal_specify=off  t_nominal_unit=N*m  t_nominal_value=1
      settings: AttributesFormatString=J in [%<inertia_unit>]
  dm : fl_lib/Mechanical/Rotational Elements/Rotational Damper  D=d_d_TMS N*m/(rad/s)  w_specify=off  w_priority=None  w=0 rad/s  w_nominal_specify=off  w_nominal_unit=rad/s  w_nominal_value=1  t_specify=off  t_priority=None  t=0 N*m  t_nominal_specify=off  t_nominal_unit=N*m  t_nominal_value=1
  Input : PMIOPort  Side=Left
  output : PMIOPort  Port=2  Side=Right
  connections:
  Rotational Spring/LConn1 -- dm/LConn1 -- Trägheitsmoment3/LConn1 -- Input/RConn1
  Rotational Spring/RConn1 -- dm/RConn1 -- output/RConn1 -- Trägheitsmoment1/LConn1

== system uz_3ph_ParameterID/Hardware/Measurement Shaft/default ==
  Trägheitsmoment3 : fl_lib/Mechanical/Rotational Elements/Inertia  inertia=d_J_Ms_M+d_J_Ms_L kg*m^2  num_ports=foundation.enum.numPorts2.one  w_specify=off  w_priority=High  w=0 rad/s  w_nominal_specify=off  w_nominal_unit=rad/s  w_nominal_value=1  t_specify=off  t_priority=None  t=0 N*m  t_nominal_specify=off  t_nominal_unit=N*m  t_nominal_value=1
      settings: AttributesFormatString=J in [%<inertia_unit>]
  Input : PMIOPort  Side=Left
  output : PMIOPort  Port=2  Side=Right
  connections:
  Trägheitsmoment3/LConn1 -- output/RConn1 -- Input/RConn1

== system uz_3ph_ParameterID/Hardware/Switch f. TMS/closed ==
  Input : PMIOPort  Side=Left
  output : PMIOPort  Port=2  Side=Right
  connections:
  output/RConn1 -- Input/RConn1

== system uz_3ph_ParameterID/Hardware/Switch f. TMS/open ==
  Rotational Free End : fl_lib/Mechanical/Rotational Elements/Rotational Free End  w_specify=off  w_priority=None  w=0 rad/s  w_nominal_specify=off  w_nominal_unit=rad/s  w_nominal_value=1
  Rotational Free End1 : fl_lib/Mechanical/Rotational Elements/Rotational Free End  w_specify=off  w_priority=None  w=0 rad/s  w_nominal_specify=off  w_nominal_unit=rad/s  w_nominal_value=1
  Input : PMIOPort  Side=Left
  output : PMIOPort  Port=2  Side=Right
  connections:
  Rotational Free End1/LConn1 -- output/RConn1
  Input/RConn1 -- Rotational Free End/LConn1

== system uz_3ph_ParameterID/Hardware/coupling m. shaft/Inertia ==
  Trägheitsmoment3 : fl_lib/Mechanical/Rotational Elements/Inertia  Commented=on  inertia=d_J_Coupling_M_Ms kg*m^2  num_ports=foundation.enum.numPorts2.one  w_specify=off  w_priority=High  w=0 rad/s  w_nominal_specify=off  w_nominal_unit=rad/s  w_nominal_value=1  t_specify=off  t_priority=None  t=0 N*m  t_nominal_specify=off  t_nominal_unit=N*m  t_nominal_value=1
      settings: AttributesFormatString=J in [%<inertia_unit>]
  Input : PMIOPort  Side=Left
  output : PMIOPort  Port=2  Side=Right
  connections:
  Input/RConn1 -- Trägheitsmoment3/LConn1 -- output/RConn1

== system uz_3ph_ParameterID/Hardware/coupling m. shaft/Spring Damper System ==
  Rotational Spring : fl_lib/Mechanical/Rotational Elements/Rotational Spring  spr_rate=d_c_Coupling_M_Ms N*m/rad  w_specify=off  w_priority=None  w=0 rad/s  w_nominal_specify=off  w_nominal_unit=rad/s  w_nominal_value=1  t_specify=off  t_priority=None  t=0 N*m  t_nominal_specify=off  t_nominal_unit=N*m  t_nominal_value=1  phi_specify=off  phi_priority=High  phi=0 rad  phi_nominal_specify=off  phi_nominal_unit=rad  phi_nominal_value=1
  Trägheitsmoment1 : fl_lib/Mechanical/Rotational Elements/Inertia  inertia=d_J_Coupling_M_Ms/2 kg*m^2  num_ports=foundation.enum.numPorts2.one  w_specify=off  w_priority=High  w=0 rad/s  w_nominal_specify=off  w_nominal_unit=rad/s  w_nominal_value=1  t_specify=off  t_priority=None  t=0 N*m  t_nominal_specify=off  t_nominal_unit=N*m  t_nominal_value=1
      settings: AttributesFormatString=J in [%<inertia_unit>]
  Trägheitsmoment3 : fl_lib/Mechanical/Rotational Elements/Inertia  inertia=d_J_Coupling_M_Ms/2 kg*m^2  num_ports=foundation.enum.numPorts2.one  w_specify=off  w_priority=High  w=0 rad/s  w_nominal_specify=off  w_nominal_unit=rad/s  w_nominal_value=1  t_specify=off  t_priority=None  t=0 N*m  t_nominal_specify=off  t_nominal_unit=N*m  t_nominal_value=1
      settings: AttributesFormatString=J in [%<inertia_unit>]
  dm : fl_lib/Mechanical/Rotational Elements/Rotational Damper  Commented=on  D=0 N*m/(rad/s)  w_specify=off  w_priority=None  w=0 rad/s  w_nominal_specify=off  w_nominal_unit=rad/s  w_nominal_value=1  t_specify=off  t_priority=None  t=0 N*m  t_nominal_specify=off  t_nominal_unit=N*m  t_nominal_value=1
  Input : PMIOPort  Side=Left
  output : PMIOPort  Port=2  Side=Right
  connections:
  Rotational Spring/LConn1 -- dm/LConn1 -- Input/RConn1 -- Trägheitsmoment3/LConn1
  Trägheitsmoment1/LConn1 -- Rotational Spring/RConn1 -- dm/RConn1 -- output/RConn1

== system uz_3ph_ParameterID/FOC/CurrentControl/id-PI-Controller with anti wind-up/Clamping circuit ==
  preSat : Inport  DisableCoverage=on  OutDataTypeStr=single
  preIntegrator : Inport  DisableCoverage=on  Port=2
  AND : Logic  DisableCoverage=on
  DataTypeConv1 : DataTypeConversion  DisableCoverage=on  OutDataTypeStr=int8  LockScale=on
  DataTypeConv2 : DataTypeConversion  DisableCoverage=on  OutDataTypeStr=int8  LockScale=on
  DeadZone : DeadZone  DisableCoverage=on  LowerValue=d_y_min  UpperValue=d_y_max
  Equal : RelationalOperator  DisableCoverage=on  Operator===
  NotEqual : RelationalOperator  DisableCoverage=on  Operator=~=
  SignDeltaU : Signum  DisableCoverage=on
  SignPreIntegrator : Signum  DisableCoverage=on
  ZeroGain : Gain  DisableCoverage=on  Gain=0  ParamDataTypeStr=double  OutDataTypeStr=single  SaturateOnIntegerOverflow=on
  Clamp : Outport  DisableCoverage=on  VectorParamsAs1DForOutWhenUnconnected=off
  wires:
  preSat/1 -> ZeroGain/1, DeadZone/1
  preIntegrator/1 -> SignPreIntegrator/1
  ZeroGain/1 -> NotEqual/1
  DeadZone/1 -> NotEqual/2, SignDeltaU/1
  SignDeltaU/1 -> DataTypeConv1/1
  DataTypeConv1/1 -> Equal/1
  SignPreIntegrator/1 -> DataTypeConv2/1
  DataTypeConv2/1 -> Equal/2
  NotEqual/1 -> AND/1
  Equal/1 -> AND/2
  AND/1 -> Clamp/1

== system uz_3ph_ParameterID/FOC/CurrentControl/iq-PI-Controller with anti wind-up/Clamping circuit ==
  preSat : Inport  DisableCoverage=on  OutDataTypeStr=single
  preIntegrator : Inport  DisableCoverage=on  Port=2
  AND : Logic  DisableCoverage=on
  DataTypeConv1 : DataTypeConversion  DisableCoverage=on  OutDataTypeStr=int8  LockScale=on
  DataTypeConv2 : DataTypeConversion  DisableCoverage=on  OutDataTypeStr=int8  LockScale=on
  DeadZone : DeadZone  DisableCoverage=on  LowerValue=d_y_min  UpperValue=d_y_max
  Equal : RelationalOperator  DisableCoverage=on  Operator===
  NotEqual : RelationalOperator  DisableCoverage=on  Operator=~=
  SignDeltaU : Signum  DisableCoverage=on
  SignPreIntegrator : Signum  DisableCoverage=on
  ZeroGain : Gain  DisableCoverage=on  Gain=0  ParamDataTypeStr=double  OutDataTypeStr=single  SaturateOnIntegerOverflow=on
  Clamp : Outport  DisableCoverage=on  VectorParamsAs1DForOutWhenUnconnected=off
  wires:
  preSat/1 -> ZeroGain/1, DeadZone/1
  preIntegrator/1 -> SignPreIntegrator/1
  ZeroGain/1 -> NotEqual/1
  DeadZone/1 -> NotEqual/2, SignDeltaU/1
  SignDeltaU/1 -> DataTypeConv1/1
  DataTypeConv1/1 -> Equal/1
  SignPreIntegrator/1 -> DataTypeConv2/1
  DataTypeConv2/1 -> Equal/2
  NotEqual/1 -> AND/1
  Equal/1 -> AND/2
  AND/1 -> Clamp/1

== system uz_3ph_ParameterID/FOC/SpeedControl/omega-PI-Controller with anti wind-up/Clamping circuit ==
  preSat : Inport  DisableCoverage=on  OutDataTypeStr=single
  preIntegrator : Inport  DisableCoverage=on  Port=2
  AND : Logic  DisableCoverage=on
  DataTypeConv1 : DataTypeConversion  DisableCoverage=on  OutDataTypeStr=int8  LockScale=on
  DataTypeConv2 : DataTypeConversion  DisableCoverage=on  OutDataTypeStr=int8  LockScale=on
  DeadZone : DeadZone  DisableCoverage=on  LowerValue=d_i_min  UpperValue=d_i_max
  Equal : RelationalOperator  DisableCoverage=on  Operator===
  NotEqual : RelationalOperator  DisableCoverage=on  Operator=~=
  SignDeltaU : Signum  DisableCoverage=on
  SignPreIntegrator : Signum  DisableCoverage=on
  ZeroGain : Gain  DisableCoverage=on  Gain=0  ParamDataTypeStr=double  OutDataTypeStr=single  SaturateOnIntegerOverflow=on
  Clamp : Outport  DisableCoverage=on  VectorParamsAs1DForOutWhenUnconnected=off
  wires:
  preSat/1 -> ZeroGain/1, DeadZone/1
  preIntegrator/1 -> SignPreIntegrator/1
  ZeroGain/1 -> NotEqual/1
  DeadZone/1 -> NotEqual/2, SignDeltaU/1
  SignDeltaU/1 -> DataTypeConv1/1
  DataTypeConv1/1 -> Equal/1
  SignPreIntegrator/1 -> DataTypeConv2/1
  DataTypeConv2/1 -> Equal/2
  NotEqual/1 -> AND/1
  Equal/1 -> AND/2
  AND/1 -> Clamp/1

== matlab function uz_3ph_ParameterID/CleanPsiArray ==
  data: OnlineID_output input; psi_array_out output; eta_c input; array_cleaned_flag output boolean; n_flux_points output
function [psi_array_out,array_cleaned_flag,n_flux_points]=clean_psi_array(OnlineID_output,eta_c)
% Author Philipp Gebhardt
% Oktober 2019

%This function is cleaning the array storing the measurement values, which always consits of a d-q-current combination a winding temperature and a speed value such as a d-q-flux combination
%The function is searching for measuring pairs which are closer than eta_c to their neighbours. In this case it is averaging these similar pairs to avoid measuring values storing the same information. 
%This is essential for calculating a wide ranging flux maps out of this array.
%Furthermore there is an output n_flux_points giving back the amount of independent measuring pairs


%Initialising Outputs
n_flux_points=single(1);
psi_array_out=single(zeros(6,100));
clean_curr_count=single(0);
array_cleaned_flag=boolean(0);

if(OnlineID_output.clean_array == 1)
% Searching for similar Datapairs
for(k=single(1):single(length(OnlineID_output.psi_array(1,:))))
    eta_count=0;
   
    if (OnlineID_output.psi_array(3,k)~=0)
        for(t=single(1):single(length(OnlineID_output.psi_array(1,:))))
            if (OnlineID_output.psi_array(3,t)~=0)
                if(k<t)    
                    if( (    (OnlineID_output.psi_array(1,k)-OnlineID_output.psi_array(1,t))^2  +...
                        (OnlineID_output.psi_array(2,k)-OnlineID_output.psi_array(2,t))^2     )^0.5 < eta_c )       
        %Averaging Datapairs if they are to close to each other
        
                        OnlineID_output.psi_array(1,t)=(OnlineID_output.psi_array(1,k)+OnlineID_output.psi_array(1,t))*0.5;
                        OnlineID_output.psi_array(2,t)=(OnlineID_output.psi_array(2,k)+OnlineID_output.psi_array(2,t))*0.5;
                        OnlineID_output.psi_array(3,t)=(OnlineID_output.psi_array(3,k)+OnlineID_output.psi_array(3,t))*0.5;
                        OnlineID_output.psi_array(4,t)=(OnlineID_output.psi_array(4,k)+OnlineID_output.psi_array(4,t))*0.5;                    
                        OnlineID_output.psi_array(5,t)=(OnlineID_output.psi_array(5,k)+OnlineID_output.psi_array(5,t))*0.5;
                        OnlineID_output.psi_array(6,t)=(OnlineID_output.psi_array(6,k)+OnlineID_output.psi_array(6,t))*0.5;     
                        OnlineID_output.psi_array(1:6,k)=0;
                        eta_count=1;  
                    end    
                end
            end
     
            if eta_count==1
                break
            end     
        end 
            if(eta_count==0)       
                %Accept values if there is enough distance between them
                clean_curr_count=clean_curr_count+1;
                psi_array_out(1,clean_curr_count)=OnlineID_output.psi_array(1,k);
                psi_array_out(2,clean_curr_count)=OnlineID_output.psi_array(2,k);
                psi_array_out(3,clean_curr_count)=OnlineID_output.psi_array(3,k);
                psi_array_out(4,clean_curr_count)=OnlineID_output.psi_array(4,k);
                psi_array_out(5,clean_curr_count)=OnlineID_output.psi_array(5,k);
                psi_array_out(6,clean_curr_count)=OnlineID_output.psi_array(6,k);
            end
    end
end

% Count flux points
for(k=single(1):single(length(psi_array_out(1,:))))  
    if(psi_array_out(1,k)~=0||psi_array_out(2,k)~=0||psi_array_out(3,k)~=0)       
           n_flux_points=k;
    end    
end

array_cleaned_flag=boolean(1);
end
return;

== matlab function uz_3ph_ParameterID/FOC/SetPoint/Field Weakening/MATLAB Function ==
  data: I_max input single; id_fw output single; ActualValues input Bus: uz_ParaID_ActualValues_t; R input single; Lq input single; Ld input single; psi_pm input single; iq_fw output; motor_type input; fw_flag output; polepairs input; M_ref input single; im_ref input single; omega_cut output
function [id_fw, iq_fw, fw_flag, omega_cut]= field_weakening(I_max, ActualValues, R, Lq, Ld, psi_pm, motor_type, polepairs, M_ref, im_ref)

fw_flag = boolean(0);
%Maximum voltage vector
u_max_dq = single(ActualValues.V_DC/sqrt(single(3)) - R*I_max)*0.95;
I1 = sqrt(ActualValues.i_dq.d^2 + ActualValues.i_dq.q^2);
%Calculation of n_cut
a = single((I1^2 * Lq^2) + psi_pm^2);
b = single(2*R*psi_pm*abs(I1));
c = single((I1^2 * R^2)-u_max_dq^2);
omega_cut = single((-b + sqrt(b^2 - 4*a*c))/(2*a));

if(M_ref ~=0)
    %Check if w_cut is valid
    if omega_cut > 0 && isreal(single(omega_cut))  
        %Calcultation of Id_ref
        if abs(ActualValues.omega_el) > omega_cut
            fw_flag = boolean(1);
            if(motor_type == 0)
                id_fw = single(psi_pm/Ld * (omega_cut/abs(ActualValues.omega_el) -1));
                id_fw = max(id_fw, -I_max);
                if(ActualValues.omega_el >0)
                    iq_fw = min(im_ref, sqrt(I_max^2 - id_fw^2));
                else
                    iq_fw = max(im_ref, -sqrt(I_max^2 - id_fw^2));
                end
            elseif(motor_type == 1)
                %Approximation with newton-raphson algorithm
                if(ActualValues.omega_el > 0)
                    iq_fw = I_max /2;
                else
                    iq_fw = -I_max /2;
                end
                c = (psi_pm^2*Lq^2 - (Ld-Lq)^2 * u_max_dq^2 / ActualValues.omega_el^2) / (Lq^2*(Ld-Lq)^2);
                d=(-4*M_ref*Ld*Lq*psi_pm)/(3*(Ld-Lq)^2*polepairs*Lq^2);
                e=((2*M_ref*Ld)^2)/(9*(Ld-Lq)^2*polepairs^2*Lq^2);

                for i=1:15
                    iq_fw = iq_fw - (iq_fw^4 + c*iq_fw^2 + d*iq_fw + e) / (4*iq_fw^3 + 2*c*iq_fw + d);
                end
                if(iq_fw <0)           
                    iq_fw = max(iq_fw, -I_max);
                else          
                    iq_fw = min(iq_fw, I_max);
                end     
                id_fw = -(psi_pm/Ld) + 1/Ld * sqrt((u_max_dq/ActualValues.omega_el)^2 - (Lq*iq_fw)^2);
            else
                id_fw = single(0);
                iq_fw = single(0.0);
            end
            id_fw = max(id_fw, -sqrt(I_max^2 - iq_fw^2));
            if id_fw > 0
                id_fw = single(0.0);
            end
        else
            id_fw = single(0.0);
            iq_fw = single(0.0);
        end
    else
        id_fw = single(0.0);
        iq_fw = single(0.0);
    end

else
    id_fw = single(0);
    iq_fw = single(0);
end

== matlab function uz_3ph_ParameterID/FOC/SetPoint/MTPA/MATLAB Function ==
  data: I_max input single; im_ref input; M_ref input; iq_ref output single; Lq input single; Ld input single; psi_pm input single; polepairs input; id_ref output; id_ref_input input; motor_type input
function [iq_ref, id_ref]= MTPA(I_max, im_ref, M_ref, Lq, Ld, psi_pm, polepairs, id_ref_input, motor_type)
if (M_ref ~= 0)
    
    if(motor_type==0)
        iq_ref = im_ref;
        id_temp = single(0);
    elseif(motor_type==1)
        %Approximation with newton-raphson algorithm
        iq_newton=im_ref;
        d=(2*M_ref*psi_pm)/(3*(Ld-Lq)^2*polepairs);
        e=((2*M_ref)^2)/(9*(Ld-Lq)^2*polepairs^2);

        for i=1:15
            iq_newton = iq_newton - (iq_newton^4 + d*iq_newton - e) / (4*iq_newton^3 + d);
        end
        if(iq_newton > 0)
            iq_ref = min(iq_newton, I_max);
        else
            iq_ref = max(iq_newton, -I_max);
        end
        if (Ld < Lq)
            id_temp = (-psi_pm / (2*(Ld - Lq))) - sqrt((psi_pm^2 / (4*(Ld - Lq)^2))+iq_ref^2 );
            id_temp = max(id_temp, -sqrt(I_max^2 - iq_ref^2));
        else
            id_temp = (-psi_pm / (2*(Ld - Lq))) + sqrt((psi_pm^2 / (4*(Ld - Lq)^2))+iq_ref^2 );
            id_temp = min(id_temp, sqrt(I_max^2 - iq_ref^2));
        end
    else
        id_temp = single(0);
        iq_ref = single(0);
    end

    id_ref = id_temp + id_ref_input;
    if(id_ref >0)
        id_ref = min(id_ref, sqrt(I_max^2 - iq_ref^2));
    else
        id_ref = max(id_ref, -sqrt(I_max^2 - iq_ref^2));
    end
else
    id_ref = single(0);
    iq_ref = single(0);
end

== matlab function uz_3ph_ParameterID/dqTrans/VoltageTransformation/Filterkorrektur_Hardware ==
  data: phi output; u input; y output; omega input; phi input

function [phi,y]= fcn(u,omega, phi)

R=95300;%ohm
RL=8200;%ohm
C=0.000000047;%Farrad
T=(RL*R*C)/(R+RL);

 w=omega;
%Filter zur Kompensation des Phasenversatz der Spannungen
 for i=single(1):single(3)
     %Rückgängigkmachen der ADC Umrechung und umkehren der Filterfunktion
u(i)=u(i)*(1+( w*T)^2)^0.5;
 end
 

phi=(phi)- atan(  w*T   );%atan(  w*T   );%*(1.08);


y = u;
